simulink model "Laboratory_2_simulink"  (R2024b)
settings: Solver=VariableStepAuto  StartTime=0.0  StopTime=10.0  RelTol=1e-3
undefined symbols (not defined in the file): b1, b2, F, k1, k2, M1, M2
settings Model: Creator=Alyssa Roca  LastModifiedBy=Alyssa Roca

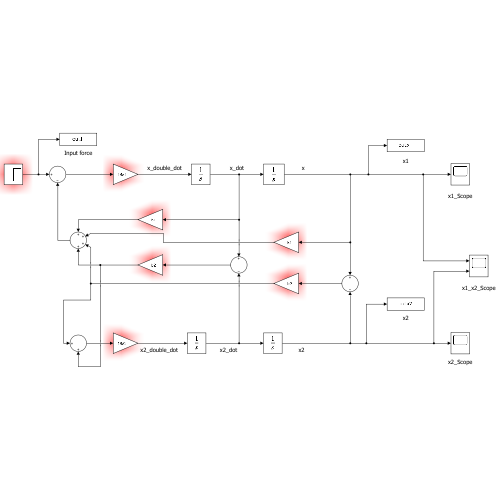
[thumbnail: Simulink's stored preview of the top-level diagram]
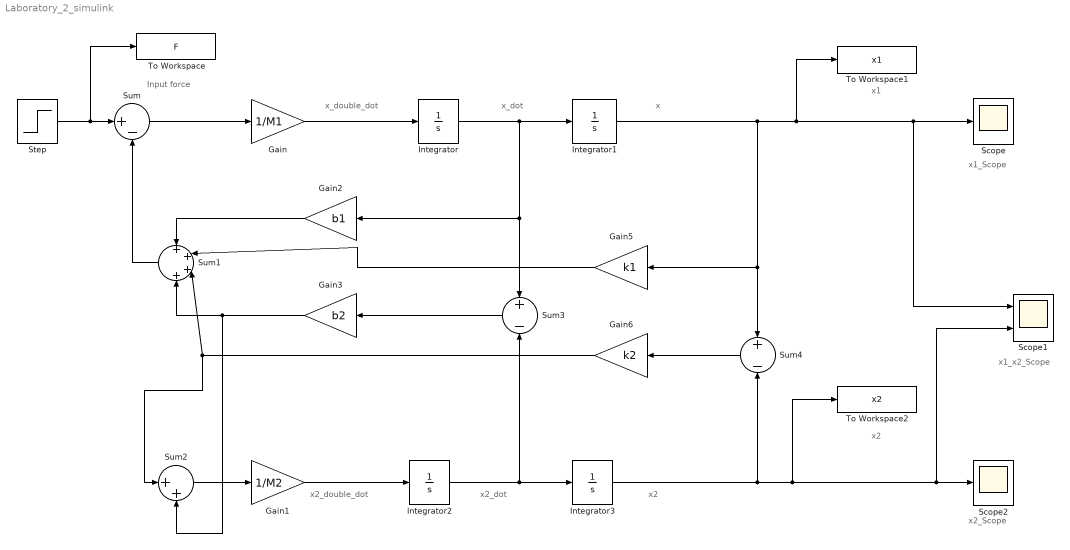
== system Laboratory_2_simulink ==
  note: x2
  note: x1_x2_Scope
  note: Input force
  note: x1
  note: x2_double_dot
  note: x_dot
  note: x2
  note: x
  note: x2_dot
  note: x_double_dot
  note: x2_Scope
  note: x1_Scope
  Gain : Gain  Gain=1/M1
  Gain1 : Gain  Gain=1/M2
  Gain2 : Gain  Gain=b1
  Gain3 : Gain  Gain=b2
  Gain5 : Gain  Gain=k1
  Gain6 : Gain  Gain=k2
  Integrator{,1..3} (4 alike) : Integrator
  Scope : Scope
  Scope1 : Scope  NumInputPorts=2
  Scope2 : Scope
  Step : Step  After=F  SampleTime=0
  Sum : Sum  Inputs=|+-
  Sum1 : Sum  Inputs=++++
  Sum2 : Sum  Inputs=|++
  Sum3 : Sum  Inputs=+-
  Sum4 : Sum  Inputs=+-
  To Workspace : ToWorkspace  VariableName=F  SaveFormat=Timeseries  SampleTime=-1
  To Workspace1 : ToWorkspace  VariableName=x1  SaveFormat=Timeseries  SampleTime=-1
  To Workspace2 : ToWorkspace  VariableName=x2  SaveFormat=Timeseries  SampleTime=-1
  wires:
  Gain3/1 -> Sum1/4, Sum2/2
  Gain1/1 -> Integrator2/1
  Gain2/1 -> Sum1/1
  Sum1/1 -> Sum/2
  Sum3/1 -> Gain3/1
  Gain6/1 -> Sum2/1, Sum1/3
  Integrator1/1 -> Gain5/1, Sum4/1, To Workspace1/1, Scope1/1, Scope/1
  Integrator2/1 -> Integrator3/1, Sum3/2
  Step/1 -> To Workspace/1, Sum/1
  Sum/1 -> Gain/1
  Integrator3/1 -> Sum4/2, To Workspace2/1, Scope1/2, Scope2/1
  Sum2/1 -> Gain1/1
  Gain/1 -> Integrator/1
  Gain5/1 -> Sum1/2
  Sum4/1 -> Gain6/1
  Integrator/1 -> Integrator1/1, Gain2/1, Sum3/1
